simulink model "diagMA_2013b"  (R2013b)
settings: Solver=ode45  SolverMode=SingleTasking  StartTime=0.0  StopTime=simTime  RelTol=1e-3
values from neighbouring files (symbols this model uses):
  alpha = 1*pi/180    (= 0.0174532925199)    [setup.m]
  b = DH/roCp    (= -11.92)    [fsolve1.m]    (also in setup.m = 7)
  c = UA/roCp/V    (= 0.3)    [fsolve1.m]    (also in setup.m = 3)
  g = 9.8    [setup.m]
  m = 1200    [setup.m]
  Ts = 0.1    [simMA.m]
  uStep = 100*g    [simMA.m]
  v0 = 0    [simMA.m]
settings Model: CovMetricSettings=dwe  CovHtmlReporting=off  covSaveCumulativeToWorkspaceVar=off  CovSaveSingleToWorkspaceVar=off  CovExternalEMLEnable=on  Creator=marcelo  LastModifiedBy=marcelo
settings DataIOCC: LimitDataPoints=off  SaveFormat=StructureWithTime
settings DebuggingCC: UnderspecifiedInitializationDetection=Simplified  MergeDetectMultiDrivingBlocksExec=error  SolverPrmCheckMsg=none  FrameProcessingCompatibilityMsg=error  SFUnexpectedBacktrackingDiag=error  SFNoUnconditionalDefaultTransitionDiag=error
settings HardwareCC: ProdBitPerPointer=64  ProdLargestAtomicFloat=Float  ProdIntDivRoundTo=Zero  ProdEndianess=LittleEndian  ProdHWDeviceType=Specified
settings ModelReferenceCC: PropagateSignalLabelsOutOfModel=on
settings SFSimCC: SimUseLocalCustomCode=on
settings RTWCC: RTWUseLocalCustomCode=on
settings GRTTargetCC: CodeReplacementLibrary=C99 (ISO)  GeneratePreprocessorConditionals=Use local settings

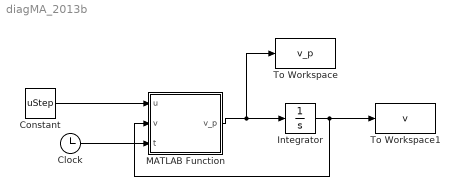
== system diagMA_2013b ==
  Clock : Clock
  Constant : Constant  Value=uStep  SampleTime=Ts
  Integrator : Integrator  InitialCondition=v0
  MATLAB Function : MATLAB Function  TreatAsAtomicUnit=on
      settings: PermitHierarchicalResolution=ParametersOnly
  To Workspace : ToWorkspace  VariableName=v_p  SaveFormat=Timeseries  SampleTime=-1
  To Workspace1 : ToWorkspace  VariableName=v  SaveFormat=Timeseries  SampleTime=-1
  wires:
  Constant/1 -> MATLAB Function/1(u)
  MATLAB Function/1(v_p) -> To Workspace/1, Integrator/1
  Integrator/1 -> To Workspace1/1, MATLAB Function/2(v)
  Clock/1 -> MATLAB Function/3(t)

== matlab function diagMA_2013b/MATLAB Function ==
  settings: updateMethod=DISCRETE  sampleTime=Ts
  data: u input; v_p output; m parameter; c parameter; g parameter; v input; alpha parameter; b parameter; t input
function v_p = fcn(u,m, c, g, v, alpha, b, t)

persistent t_OLD; % declaração da variável persistente (que retém o
                  %valor da última iteração

if isempty(t_OLD) % inicialização
    t_OLD = 0;
end

v_p = (1/m)*(u - b*v - c*(v^2) - m*g*sin(alpha));

Dt = t - t_OLD; %(exemplo) cálculo do período de amostragem desta função

t_OLD = t; % atualização da variável persistente

end
